simulink model "coverage2D"  (R2024a)
settings: Solver=ode1  StartTime=0.0  StopTime=Tf  FixedStep=step_size  MaxStep=0.01  MinStep=0.001  RelTol=1e-3
values from neighbouring files (symbols this model uses):
  a = [100 amin*ones(1,7) 100]'    [coverage2D_parameters.m]
  a_hat0 = amin * ones(9,n)    [coverage2D_parameters.m]
  amin = 0.1    [coverage2D_parameters.m]
  g = 100    [coverage2D_parameters.m]
  Gamma = eye(9)    [coverage2D_parameters.m]
  K = [3 3; -3 3]    [coverage2D_parameters.m]
  Li0 = Li0(:)    [coverage2D_parameters.m]
  li0 = zeros(9,n)    [coverage2D_parameters.m]
  n = 20    [coverage2D_parameters.m]    (also in phi_heatmap.m = 100)
  p0 = [x0, y0]    [coverage2D_parameters.m]
  psi = 0    [coverage2D_parameters.m]
  step_size = 0.01    [coverage2D_parameters.m]
settings Model: SimulationMode=accelerator  Creator=valen  LastModifiedBy=valen
settings SolverCC: ShapePreserveControl=EnableAll  ODENIntegrationMethod=ode1

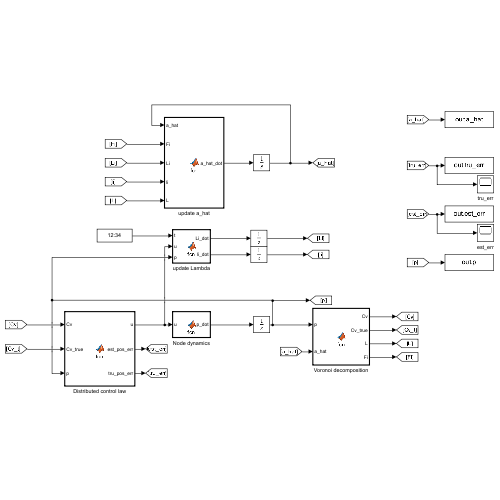
[thumbnail: Simulink's stored preview of the top-level diagram]
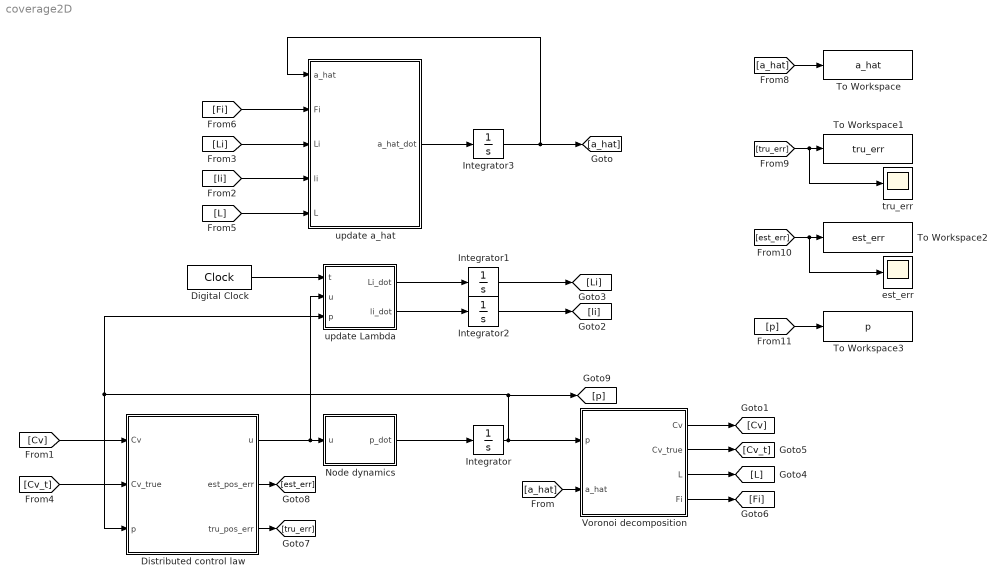
== system coverage2D ==
  Digital Clock : DigitalClock  SampleTime=step_size
  Distributed control law : MATLAB Function  TreatAsAtomicUnit=on
  Integrator : Integrator  InitialCondition=p0
  Integrator1 : Integrator  InitialCondition=Li0
  Integrator2 : Integrator  InitialCondition=li0
  Integrator3 : Integrator  InitialCondition=a_hat0
  Node dynamics : MATLAB Function  TreatAsAtomicUnit=on
  To Workspace : ToWorkspace  VariableName=a_hat  SaveFormat=Timeseries  SampleTime=-1
  To Workspace1 : ToWorkspace  VariableName=tru_err  SaveFormat=Timeseries  SampleTime=-1
  To Workspace2 : ToWorkspace  VariableName=est_err  SaveFormat=Timeseries  SampleTime=-1
  To Workspace3 : ToWorkspace  VariableName=p  SaveFormat=Timeseries  SampleTime=-1
  Voronoi decomposition : MATLAB Function  TreatAsAtomicUnit=on
  est_err : Scope
  tru_err : Scope
  update Lambda : MATLAB Function  TreatAsAtomicUnit=on
  update a_hat : MATLAB Function  TreatAsAtomicUnit=on
  wires:
  Node dynamics/1(p_dot) -> Integrator/1
  Distributed control law/1(u) -> update Lambda/2(u), Node dynamics/1(u)
  update Lambda/2(li_dot) -> Integrator2/1
  update Lambda/1(Li_dot) -> Integrator1/1
  update a_hat/1(a_hat_dot) -> Integrator3/1
  Integrator3/1 -> update a_hat/1(a_hat), [a_hat]
  [a_hat] -> Voronoi decomposition/2(a_hat)
  Voronoi decomposition/1(Cv) -> [Cv]
  [Cv] -> Distributed control law/1(Cv)
  Integrator/1 -> update Lambda/3(p), Distributed control law/3(p), [p], Voronoi decomposition/1(p)
  Integrator2/1 -> [li]
  Integrator1/1 -> [Li]
  [li] -> update a_hat/4(li)
  [Li] -> update a_hat/3(Li)
  Voronoi decomposition/3(L) -> [L]
  Voronoi decomposition/2(Cv_true) -> [Cv_t]
  [Cv_t] -> Distributed control law/2(Cv_true)
  [L] -> update a_hat/5(L)
  Voronoi decomposition/4(Fi) -> [Fi]
  [Fi] -> update a_hat/2(Fi)
  Distributed control law/2(est_pos_err) -> [est_err]
  Distributed control law/3(tru_pos_err) -> [tru_err]
  [a_hat] -> To Workspace/1
  [tru_err] -> tru_err/1, To Workspace1/1
  [est_err] -> est_err/1, To Workspace2/1
  [p] -> To Workspace3/1
  Digital Clock/1 -> update Lambda/1(t)

== matlab function coverage2D/Voronoi decomposition ==
  data: p input; Cv output; a_hat input; Cv_true output; L output; Fi output; n parameter
function [Cv, Cv_true, L, Fi] = fcn(p, a_hat,n)
    coder.extrinsic('VoronoiDecomposition');

    % preallocation for interpreted matlab functions
    Cv = zeros(2,n);
    Cv_true = zeros(2,n);
    L = zeros(n,n);
    Fi = zeros(9,9,n);
    
    [Cv, Cv_true, L, Fi] = VoronoiDecomposition(p, a_hat);

end

== matlab function coverage2D/Node dynamics ==
  data: u input; p_dot output
function p_dot = fcn(u)

    p_dot = u;
end

== matlab function coverage2D/Distributed control law ==
  data: Cv input; Cv_true input; u output; p input; est_pos_err output; tru_pos_err output; K parameter
function [u, est_pos_err, tru_pos_err] = fcn(Cv,Cv_true, p, K)
    px = p(:,1);
    py = p(:,2);

    ux = K(1,1)*(Cv(1,:)' - px);
    uy = K(2,2)*(Cv(2,:)' - py);
    
    u = [ux, uy];

    est_pos_err = mean(vecnorm([(Cv(1,:)' - px),(Cv(2,:)' - py)]'));
    tru_pos_err = mean(vecnorm([(Cv_true(1,:)' - px),(Cv_true(2,:)' - py)]'));

== matlab function coverage2D/update Lambda ==
  data: t input; u input; p input; Li_dot output; li_dot output; n parameter; K parameter; a parameter
function [Li_dot, li_dot] = fcn(t, u, p, n, K, a)
    
    coder.extrinsic('kappa');

    ux = u(:,1);
    uy = u(:,2);

    px = p(:,1);
    py = p(:,2);

    li_dot = zeros(9, n);
    Li_dot_ = zeros(9,9,n);
    for i = 1:n

        if t>10
            w_t = 0;
        else
            w_t = norm([ux(i) uy(i)])^2/norm(K)^2; % Data weighting function
        end
        ki = kappa(px(i),py(i));
        phi_t = ki*a;
        Li_dot_(:,:,i) = w_t*(ki'*ki);
        li_dot(:,i) = w_t*(phi_t)*ki';
    end

    Li_dot = Li_dot_(:);

== matlab function coverage2D/update a_hat ==
  data: a_hat input; a_hat_dot output; Fi input; Li input; li input; L input; psi parameter; g parameter; n parameter; Gamma parameter; amin parameter; step_size parameter
function a_hat_dot = fcn(a_hat, Fi, Li, li, L, psi, g, n, Gamma, amin, step_size)

% Reshape back from integrator
Li = reshape(Li, 9, 9, n);
a_hat_dot = zeros(size(a_hat));

% Adaption laws for paramter estimate
s = a_hat*L';
for i = 1:n
    ai_hat_dot = -(Fi(:,:,i)*a_hat(:,i)) - g*(Li(:,:,i)*a_hat(:,i) - li(:,i)) - psi*s(:,i);

    % prevent a_hat to become zero
    Iproji = zeros(9,1);
    Iproji(a_hat(:,i) + ai_hat_dot*step_size <= amin) = 1;
    
    a_hat_dot(:,i) = Gamma*(ai_hat_dot - diag(Iproji)*ai_hat_dot);    
end
